simulink model "body_model"  (R2018b)
settings: Solver=VariableStepAuto  StartTime=0.0  StopTime=10.0  RelTol=1e-3
InitFcn:
  | %Robot_Body_Constants
values from neighbouring files (symbols this model uses):
  robot_mass = 0.743    [Robot_Body_Constants.m]
  robot_radius = 0.0789    [Robot_Body_Constants.m]
settings Model: Creator=Zach  LastModifiedBy=Zach

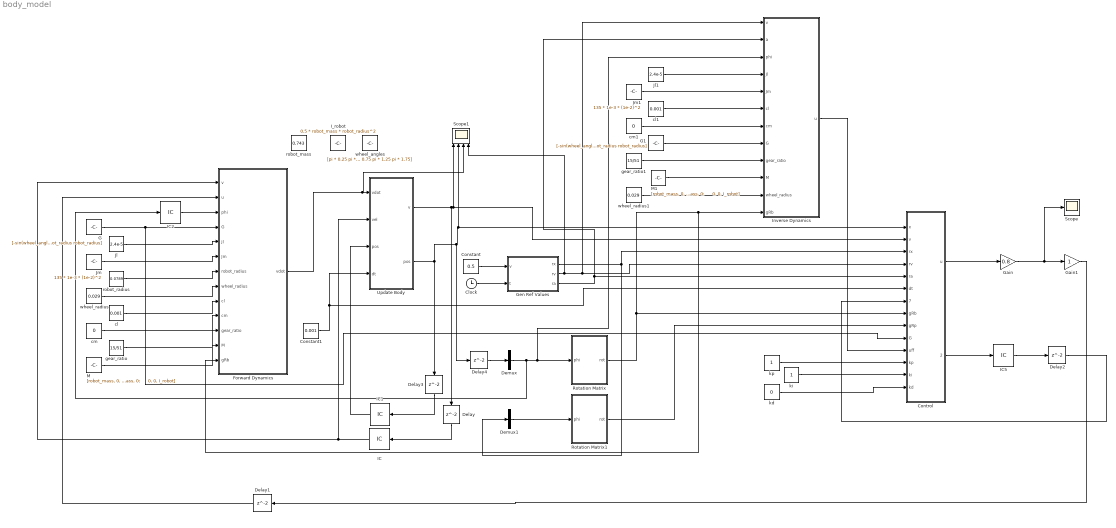
== system body_model ==
  Clock : Clock
  Constant : Constant  Value=0.5
  Constant1 : Constant  Value=0.001
  Control : MATLAB Function  TreatAsAtomicUnit=on
  Delay{,1..4} (5 alike) : Delay
  Demux : Demux  Outputs=3
  Demux1 : Demux  Outputs=3
  Forward Dynamics : MATLAB Function  TreatAsAtomicUnit=on
  G : Constant  Value=|
      | [-sin(wheel_angles(1)) -sin(wheel_angles(2)) -sin(wheel_angles(3)) -sin(wheel_angles(4));
      |      cos(wheel_angles(1)) cos(wheel_angles(2)) cos(wheel_angles(3)) cos(wheel_angles(4));
      |      robot_radius robot_radius robot_radius robot_radius]
  G1 : Constant  Value=|
      | [-sin(wheel_angles(1)) -sin(wheel_angles(2)) -sin(wheel_angles(3)) -sin(wheel_angles(4));
      |      cos(wheel_angles(1)) cos(wheel_angles(2)) cos(wheel_angles(3)) cos(wheel_angles(4));
      |      robot_radius robot_radius robot_radius robot_radius]
  Gain : Gain  Gain=0.8
  Gain1 : Gain
  Gen Ref Values : MATLAB Function  TreatAsAtomicUnit=on
  IC : InitialCondition  Value=[0 0 0]'
  IC1 : InitialCondition  Value=[0 0 0]
  IC2 : InitialCondition  Value=0
  IC5 : InitialCondition  Value=[0 0 0]
  I_robot : Constant  Value=0.5 * robot_mass * robot_radius^2
  Inverse Dynamics : MATLAB Function  TreatAsAtomicUnit=on
  Jl : Constant  Value=2.4e-5
  Jl1 : Constant  Value=2.4e-5
  Jm : Constant  Value=135 * 1e-3 * (1e-2)^2
  Jm1 : Constant  Value=135 * 1e-3 * (1e-2)^2
  M : Constant  Value=|
      | [robot_mass, 0, 0;
      |      0, robot_mass, 0;
      |      0, 0, I_robot]
  M1 : Constant  Value=|
      | [robot_mass, 0, 0;
      |      0, robot_mass, 0;
      |      0, 0, I_robot]
  Rotation Matrix : MATLAB Function  TreatAsAtomicUnit=on
  Rotation Matrix1 : MATLAB Function  TreatAsAtomicUnit=on
  Scope : Scope
  Scope1 : Scope  NumInputPorts=4
  Update Body : MATLAB Function  TreatAsAtomicUnit=on
  cl : Constant  Value=0.001
  cl1 : Constant  Value=0.001
  cm : Constant  Value=0
  cm1 : Constant  Value=0
  gear_ratio : Constant  Value=15/51
  gear_ratio1 : Constant  Value=15/51
  kd : Constant  Value=0
  ki : Constant
  kp : Constant
  robot_mass : Constant  Value=0.743
  robot_radius : Constant  Value=0.0789
  wheel_angles : Constant  Value=[pi * 0.25 pi * 0.75 pi * 1.25 pi * 1.75]
  wheel_radius : Constant  Value=0.029
  wheel_radius1 : Constant  Value=0.029
  wires:
  Update Body/2(pos) -> Delay4/1, Control/1(x), Scope1/2, Delay3/1
  IC2/1 -> Forward Dynamics/3(phi)
  Forward Dynamics/1(vdot) -> Scope1/3, Update Body/1(vdot)
  Clock/1 -> Gen Ref Values/2(t)
  G/1 -> Control/10(G), Forward Dynamics/4(G)
  Jl/1 -> Forward Dynamics/5(Jl)
  Jm/1 -> Forward Dynamics/6(Jm)
  robot_radius/1 -> Forward Dynamics/7(robot_radius)
  gear_ratio/1 -> Forward Dynamics/11(gear_ratio)
  M/1 -> Forward Dynamics/12(M)
  cm/1 -> Forward Dynamics/10(cm)
  cl/1 -> Forward Dynamics/9(cl)
  wheel_radius/1 -> Forward Dynamics/8(wheel_radius)
  Control/2(integral) -> IC5/1
  IC5/1 -> Delay2/1
  Delay2/1 -> Control/7("integral ")
  Gen Ref Values/1(rx) -> Demux1/1, Control/3(rx)
  Gen Ref Values/2(rv) -> Inverse Dynamics/1(v), Control/4(rv), Scope1/4
  Gen Ref Values/3(ra) -> Inverse Dynamics/2(a), Control/5(ra)
  Control/1(u) -> Gain/1
  Update Body/1(v) -> Control/2(v), Scope1/1, Delay/1
  Constant/1 -> Gen Ref Values/1(v)
  IC/1 -> Update Body/2(vel), Forward Dynamics/1(v)
  Delay/1 -> IC/1
  Gain/1 -> Gain1/1, Scope/1
  Gain1/1 -> Delay1/1
  Delay1/1 -> Forward Dynamics/2(u)
  Constant1/1 -> Update Body/4(dt), Control/6(dt)
  Delay3/1 -> IC1/1
  IC1/1 -> Update Body/3("pos ")
  Rotation Matrix/1(rot) -> Forward Dynamics/13(gRb), Inverse Dynamics/12(gRb), Control/8(gRb)
  Demux/2 -> IC2/1, Inverse Dynamics/3(phi), Rotation Matrix/1(phi)
  Rotation Matrix1/1(rot) -> Control/9(gRp)
  Demux1/2 -> Rotation Matrix1/1(phi)
  Jm1/1 -> Inverse Dynamics/5(Jm)
  G1/1 -> Inverse Dynamics/8(G)
  Jl1/1 -> Inverse Dynamics/4(Jl)
  cl1/1 -> Inverse Dynamics/6(cl)
  cm1/1 -> Inverse Dynamics/7(cm)
  gear_ratio1/1 -> Inverse Dynamics/9(gear_ratio)
  M1/1 -> Inverse Dynamics/10(M)
  wheel_radius1/1 -> Inverse Dynamics/11(wheel_radius)
  Inverse Dynamics/1(u) -> Control/11(uff)
  kp/1 -> Control/12(kp)
  ki/1 -> Control/13(ki)
  kd/1 -> Control/14(kd)
  Delay4/1 -> Demux/1

== matlab function body_model/Gen Ref Values ==
  data: v input; rx output; t input; rv output; ra output
function [rx, rv, ra] = update_control(v,t)
    rx = [sin(v * t); cos(v * t); v * t];
    rv = v * [cos(v * t); -sin(v * t); v];
    ra = v^2 * [-sin(v * t); -cos(v * t); 0];

%    u = 0.8 * robot_controller.control(pos, vel, rx, rv, ra);
end

== matlab function body_model/Control ==
  data: x input; v input; rx input; rv input; ra input; dt input; u output; integral input; integral output; gRb input; gRp input; G input; uff input; kp input; ki input; kd input
function [u, integral] = control(x, v, rx, rv, ra, dt, integral, gRb, gRp, G, uff, kp, ki, kd)
    %gRb = rotation_matrix(x(2));
    %gRp = rotation_matrix(rx(2));
    error_path_relative = gRp * (rx - x);
    integral = integral + (dt * [1 0 0; 0 1 0; 0 0 1e-2] \ error_path_relative);

    Ginv = pinv(G);
    error = gRb' * (rx - x);
    error(3, 1) = error(3, 1) * 0.1;

    derivative = gRb' * (rv - v);
    derivative(3, 1) = derivative(3, 1) * 0.01;

    %uff = inverse_dynamics(rv, ra, x(2));%call inverse_dynamics
    up = kp * Ginv * error;
    ui = ki * Ginv * gRb * gRp' * integral;
    ud = kd * Ginv * derivative;

    u = uff + up + ui + ud;
end

== matlab function body_model/Update Body ==
  data: vdot input; vel input; v output; pos input; dt input; pos output
function [v,pos] = update_body(vdot, vel, pos, dt)

pos = pos + (dt * vel) + (0.5 * vdot * dt^2);
v = (dt * vdot);

== matlab function body_model/Rotation Matrix ==
  data: phi input; rot output
function rot = rotation_matrix(phi)
    rot = [cos(phi) -sin(phi) 0; sin(phi) cos(phi) 0; 0 0 1];
end

== matlab function body_model/Rotation Matrix1 ==
  data: phi input; rot output
function rot = rotation_matrix(phi)
    rot = [cos(phi) -sin(phi) 0; sin(phi) cos(phi) 0; 0 0 1];
end

== matlab function body_model/Inverse Dynamics ==
  data: v input; u output; a input; phi input; Jl input; Jm input; cl input; cm input; G input; gear_ratio input; M input; wheel_radius input; gRb input
function u = inverse_dynamics(v, a, phi, Jl, Jm, cl, cm, G, gear_ratio, M, wheel_radius, gRb)
    phidot = v(3, 1); %Double check this
    I4 = eye(4);
    GTinv = pinv(G');
    Ginv = pinv(G);
    %gRb = rotation_matrix(phi);
    w_l = G' * gRb' * v / wheel_radius;
    
    Rdot = -phidot * [-sin(phi), -cos(phi), 0; cos(phi), sin(phi), 0; 0, 0, 0];
    RTRdot = phidot * [0 1 0; -1 0 0; 0 0 0];
    
    Z = (((Jm + Jl) / gear_ratio^2) * I4) + (wheel_radius^2/gear_ratio^2) * (Ginv * M) * GTinv;
    v = ((cm + cl / gear_ratio^2) * I4) + (wheel_radius^2/gear_ratio^2) * (Ginv * RTRdot) * GTinv;
    
    wldot = (G' * gRb' / wheel_radius) * (a - Rdot * GTinv * wheel_radius * w_l);
    A = -pinv(Z) * v;
    u = Z * gear_ratio * (wldot - A * w_l);
end

== matlab function body_model/Forward Dynamics ==
  data: v input; u input; vdot output; phi input; G input; Jl input; Jm input; robot_radius input; wheel_radius input; cl input; cm input; gear_ratio input; M input; gRb input
 function vdot = forward_dynamics(v, u, phi, G, Jl, Jm, robot_radius, wheel_radius, cl, cm, gear_ratio, M, gRb)
    phidot = v(3, 1); %Double check this
    I4 = eye(4);
    GTinv = pinv(G');
    Ginv = pinv(G);
   % gRb = rotation_matrix(phi);
    w_l = G' * gRb' * v / robot_radius;
    
    Rdot = -phidot * [-sin(phi), -cos(phi), 0; cos(phi), sin(phi), 0; 0, 0, 0];
    RTRdot = phidot * [0 1 0; -1 0 0; 0 0 0];
    
    Z = (((Jm + Jl) / gear_ratio^2) * I4) + (wheel_radius^2/gear_ratio^2) * Ginv * M * GTinv;
    V = ((cm + cl / gear_ratio^2) * I4) + (wheel_radius^2/gear_ratio^2) * Ginv * RTRdot * GTinv;
    
    B = pinv(Z)/gear_ratio;
    A = pinv(Z) * V;
    wldot = A * w_l + B * u;
    
    vdot = Rdot * GTinv * wheel_radius * w_l + gRb * GTinv * wheel_radius * wldot;
end
